simulink model "ZeroCrossingSimple"  (R2022b)
settings: Solver=FixedStepDiscrete  StartTime=0.0  StopTime=0.08  FixedStep=1e-6  RelTol=1e-3
libraries: simulink x2
settings Model: Creator=ahmed  LastModifiedBy=ahmed

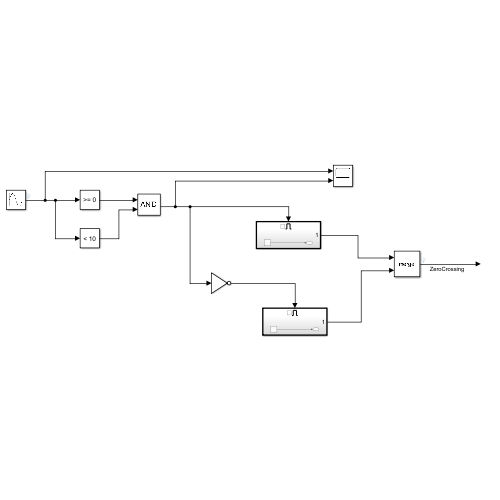
[thumbnail: Simulink's stored preview of the top-level diagram]
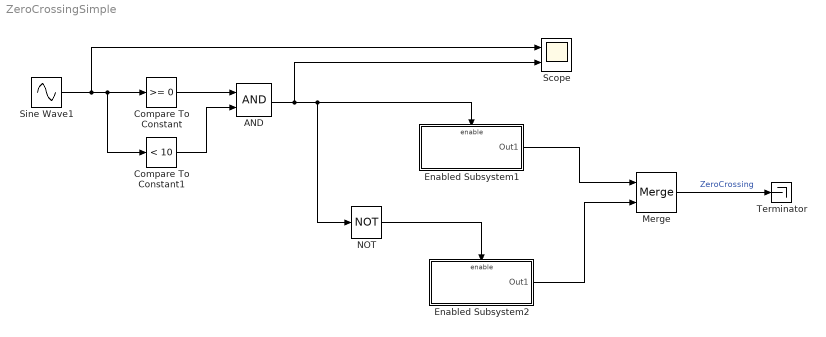
== system ZeroCrossingSimple ==
  AND : Logic  AllPortsSameDT=off  OutDataTypeStr=boolean
  Compare To Constant : simulink/Logic and Bit Operations/Compare To Constant  relop=>=  const=0  OutDataTypeStr=boolean
  Compare To Constant1 : simulink/Logic and Bit Operations/Compare To Constant  relop=<  const=10  OutDataTypeStr=boolean
  Enabled Subsystem1 : Subsystem  TreatAsAtomicUnit=on
  Enabled Subsystem2 : Subsystem  TreatAsAtomicUnit=on
  Merge : Merge
  NOT : Logic  Operator=NOT  IconShape=distinctive  AllPortsSameDT=off  OutDataTypeStr=boolean
  Scope : Scope  NumInputPorts=2
  Sine Wave1 : Sin  Amplitude=220  Frequency=2*pi*50  SampleTime=0
  Terminator : Terminator
  wires:
  Sine Wave1/1 -> Scope/1, Compare To Constant1/1, Compare To Constant/1
  Compare To Constant/1 -> AND/1
  Compare To Constant1/1 -> AND/2
  AND/1 -> Scope/2, NOT/1, Enabled Subsystem1/Enable
  NOT/1 -> Enabled Subsystem2/Enable
  Enabled Subsystem1/1(Out1) -> Merge/1
  Enabled Subsystem2/1(Out1) -> Merge/2
  Merge/1 -> Terminator/1  "ZeroCrossing"

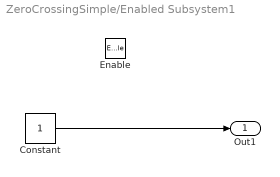
== system ZeroCrossingSimple/Enabled Subsystem1 ==
  Enable : EnablePort
  Constant : Constant
  Out1 : Outport
  wires:
  Constant/1 -> Out1/1

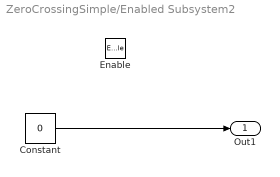
== system ZeroCrossingSimple/Enabled Subsystem2 ==
  Enable : EnablePort
  Constant : Constant  Value=0
  Out1 : Outport
  wires:
  Constant/1 -> Out1/1
